simulink model "pmsm_model_Lab3_MTPA_st_R2020a"  (R2023a)
settings: Solver=ode45  StartTime=0.0  StopTime=Tf  FixedStep=Tsim  MaxStep=Tsim  MinStep=Tsim/100  RelTol=1e-3
values from neighbouring files (symbols this model uses):
  C32 = [ 1       0 ... (first row only)    [pmsm_param_Lab1_2025.m]    (also in pmsm_param_Lab2_2025_st.m; pmsm_param_Lab3_st.m; pmsm_param_Lab4_2024_st.m)
  C32inv = 2/3*[1    -1/2        -1/2 ... (first row only)    [pmsm_param_Lab1_2025.m]    (also in pmsm_param_Lab2_2025_st.m; pmsm_param_Lab3_st.m; pmsm_param_Lab4_2024_st.m)
  C33 = C32*C32inv    [pmsm_param_Lab1_2025.m]    (also in pmsm_param_Lab2_2025_st.m; pmsm_param_Lab3_st.m; pmsm_param_Lab4_2024_st.m)
  Cb = 500e-6    (= 0.0005)    [pmsm_param_Lab3_st.m]    (also in pmsm_param_Lab4_2024_st.m)
  dTm0 = 0.20*Tmrated    (= 48)    [pmsm_param_Lab2_2025_st.m]    (also in pmsm_param_Lab3_st.m; pmsm_param_Lab4_2024_st.m = 120)
  Dyno = 1    [pmsm_param_Lab3_st.m]    (also in pmsm_param_Lab4_2024_st.m = 0)
  f = 15e-3    (= 0.015)    [pmsm_param_Lab1_2025.m]    (also in pmsm_param_Lab2_2025_st.m; pmsm_param_Lab3_st.m; pmsm_param_Lab4_2024_st.m)
  GVSI = 1    [pmsm_param_Lab2_2025_st.m]    (also in pmsm_param_Lab3_st.m; pmsm_param_Lab4_2024_st.m)
  Id0 = 0    [pmsm_param_Lab1_2025.m]    (also in pmsm_param_Lab2_2025_st.m; pmsm_param_Lab3_st.m = interp1(Tref,Idopt,Tm0); pmsm_param_Lab4_2024_st.m = interp1(Tref,Idopt,Tm0))
  Idc0 = Pe0/VDC    [pmsm_param_Lab3_st.m]    (also in pmsm_param_Lab4_2024_st.m)
  Idopt = zeros(1,NT)    [pmsm_param_Lab3_st.m]    (also in pmsm_param_Lab4_2024_st.m)
  Iq0 = 2/3*Tm0/(Pp*Psif)    (= 0)    [pmsm_param_Lab1_2025.m]    (also in pmsm_param_Lab2_2025_st.m = 119.926066866; pmsm_param_Lab3_st.m = interp1(Tref,Iqopt,Tm0); pmsm_param_Lab4_2024_st.m = interp1(Tref,Iqopt,Tm0))
  Iqopt = zeros(1,NT)    [pmsm_param_Lab3_st.m]    (also in pmsm_param_Lab4_2024_st.m)
  J = 100e-3    (= 0.1)    [pmsm_param_Lab1_2025.m]    (also in pmsm_param_Lab2_2025_st.m; pmsm_param_Lab3_st.m; pmsm_param_Lab4_2024_st.m)
  Kid = Kpd / tid    (= 282.743237724)    [pmsm_param_Lab2_2025_st.m]    (also in pmsm_param_Lab3_st.m = 180; pmsm_param_Lab4_2024_st.m = 180)
  Kiq = Kpq / tiq    (= 282.743237724)    [pmsm_param_Lab2_2025_st.m]    (also in pmsm_param_Lab3_st.m = 180; pmsm_param_Lab4_2024_st.m = 180)
  kL = 0.750    (= 0.75)    [pmsm_param_Lab1_2025.m]    (also in pmsm_param_Lab2_2025_st.m; pmsm_param_Lab3_st.m; pmsm_param_Lab4_2024_st.m)
  Kpd = (3*Ld0) / tr    (= 6.28318306054)    [pmsm_param_Lab2_2025_st.m]    (also in pmsm_param_Lab3_st.m = 3; pmsm_param_Lab4_2024_st.m = 3)
  Kpq = (3 * Lq0) / tr    (= 3.14159153027)    [pmsm_param_Lab2_2025_st.m]    (also in pmsm_param_Lab3_st.m = 6; pmsm_param_Lab4_2024_st.m = 6)
  Lb = 20e-6    (= 2e-05)    [pmsm_param_Lab3_st.m]    (also in pmsm_param_Lab4_2024_st.m)
  Ld0 = 2.0*Ld    (= 0.002)    [pmsm_param_Lab2_2025_st.m]    (also in pmsm_param_Lab3_st.m = 0.001; pmsm_param_Lab4_2024_st.m = 0.001)
  Lq0 = 0.5*Lq    (= 0.001)    [pmsm_param_Lab2_2025_st.m]    (also in pmsm_param_Lab3_st.m = 0.002; pmsm_param_Lab4_2024_st.m = 0.002)
  Pe0 = 3/2*(Vd0*Id0+Vq0*Iq0)    [pmsm_param_Lab2_2025_st.m]    (also in pmsm_param_Lab3_st.m; pmsm_param_Lab4_2024_st.m)
  Pp = 4    [pmsm_param_Lab1_2025.m]    (also in pmsm_param_Lab2_2025_st.m; pmsm_param_Lab3_st.m; pmsm_param_Lab4_2024_st.m)
  Psid0 = interpn(Idv,Iqv,Psidd,Id0,Iq0)    [pmsm_param_Lab1_2025.m]    (also in pmsm_param_Lab2_2025_st.m; pmsm_param_Lab3_st.m; pmsm_param_Lab4_2024_st.m)
  Psif0 = 1.0*Psif    (= 0.167)    [pmsm_param_Lab2_2025_st.m]    (also in pmsm_param_Lab3_st.m; pmsm_param_Lab4_2024_st.m)
  Psiq0 = interpn(Idv,Iqv,Psiqq,Id0,Iq0)    [pmsm_param_Lab1_2025.m]    (also in pmsm_param_Lab2_2025_st.m; pmsm_param_Lab3_st.m; pmsm_param_Lab4_2024_st.m)
  Qbat = 72*3600    (= 259200)    [pmsm_param_Lab3_st.m]    (also in pmsm_param_Lab4_2024_st.m)
  RateTm = 10000    [pmsm_param_Lab3_st.m]    (also in pmsm_param_Lab4_2024_st.m)
  rb = 80e-3    (= 0.08)    [pmsm_param_Lab3_st.m]    (also in pmsm_param_Lab4_2024_st.m)
  Rs = 60e-3    (= 0.06)    [pmsm_param_Lab1_2025.m]    (also in pmsm_param_Lab2_2025_st.m; pmsm_param_Lab3_st.m; pmsm_param_Lab4_2024_st.m)
  Rs0 = 1.5*Rs    (= 0.09)    [pmsm_param_Lab2_2025_st.m]    (also in pmsm_param_Lab3_st.m = 0.06; pmsm_param_Lab4_2024_st.m = 0.06)
  SOC0 = 0.50    (= 0.5)    [pmsm_param_Lab3_st.m]    (also in pmsm_param_Lab4_2024_st.m)
  Thetae0 = 0    [pmsm_param_Lab1_2025.m]    (also in pmsm_param_Lab2_2025_st.m; pmsm_param_Lab3_st.m; pmsm_param_Lab4_2024_st.m)
  Tm0 = (kL+f)*Wm0    (= 0)    [pmsm_param_Lab1_2025.m]    (also in pmsm_param_Lab2_2025_st.m = 120.165919; pmsm_param_Lab3_st.m = 192.2654704; pmsm_param_Lab4_2024_st.m)
  Tp = 100e-6    (= 0.0001)    [pmsm_param_Lab2_2025_st.m]    (also in pmsm_param_Lab3_st.m; pmsm_param_Lab4_2024_st.m)
  Tref = -Tmax:Tmax/100:Tmax    [pmsm_param_Lab3_st.m]    (also in pmsm_param_Lab4_2024_st.m)
  Ts = Tsim    [pmsm_param_Lab2_2025_st.m]    (also in pmsm_param_Lab3_st.m = 0.0001; pmsm_param_Lab4_2024_st.m = 0.0001)
  Tsim = 1e-6    (= 1e-06)    [pmsm_param_Lab1_2025.m]    (also in pmsm_param_Lab2_2025_st.m = min([Tp Ts])/100; pmsm_param_Lab3_st.m = min([Tp Ts])/100; pmsm_param_Lab4_2024_st.m = min([Tp Ts])/100)
  TSS = Tstep+0.050    (= 0.1)    [pmsm_param_Lab3_st.m]    (also in pmsm_param_Lab4_2024_st.m)
  Tstep = 0.10    (= 0.1)    [pmsm_param_Lab2_2025_st.m]    (also in pmsm_param_Lab3_st.m = 0.05; pmsm_param_Lab4_2024_st.m = 0.05)
  Ud0 = Rs*Id0    (= 0)    [pmsm_param_Lab2_2025_st.m]    (also in pmsm_param_Lab3_st.m; pmsm_param_Lab4_2024_st.m)
  Uq0 = Rs*Iq0    (= 7.19556401196)    [pmsm_param_Lab2_2025_st.m]    (also in pmsm_param_Lab3_st.m = 11.5129024191; pmsm_param_Lab4_2024_st.m = Rs*Iq0)
  Vd0 = Rs*Id0-Pp*Psiq0*Wm0    [pmsm_param_Lab1_2025.m]    (also in pmsm_param_Lab2_2025_st.m = Ud0-Pp*Psiq0*Wm0; pmsm_param_Lab3_st.m = Ud0-Pp*Psiq0*Wm0; pmsm_param_Lab4_2024_st.m = Ud0-Pp*Psiq0*Wm0)
  VDC = 800    [pmsm_param_Lab2_2025_st.m]    (also in pmsm_param_Lab3_st.m; pmsm_param_Lab4_2024_st.m)
  VDC0 = 0.8*VDC    (= 640)    [pmsm_param_Lab3_st.m]    (also in pmsm_param_Lab4_2024_st.m)
  Vp = VDC/2    (= 400)    [pmsm_param_Lab2_2025_st.m]    (also in pmsm_param_Lab3_st.m; pmsm_param_Lab4_2024_st.m)
  Vq0 = Rs*Iq0+Pp*Psid0*Wm0    [pmsm_param_Lab1_2025.m]    (also in pmsm_param_Lab2_2025_st.m = Uq0+Pp*Psid0*Wm0; pmsm_param_Lab3_st.m = Uq0+Pp*Psid0*Wm0; pmsm_param_Lab4_2024_st.m = Uq0+Pp*Psid0*Wm0)
  Wm0 = 0    [pmsm_param_Lab1_2025.m]    (also in pmsm_param_Lab2_2025_st.m = 157.079632679; pmsm_param_Lab3_st.m = 251.327412287; pmsm_param_Lab4_2024_st.m)
undefined symbols (not defined in the file or in its folder): Idd, Idrop, Iqq, Isw, Psidv, Psiqv, SwLoss, Vdrop
libraries: simulink x11, spsTHDLib x1
(part 1 of 2)
settings Model: Creator=babak_  LastModifiedBy=Henry
settings SolverCC: AlgebraicLoopSolver=LineSearch
settings DataIOCC: LimitDataPoints=on  SaveFormat=Array  SignalLoggingSaveFormat=ModelDataLogs  ReturnWorkspaceOutputs=off
settings OptimizationCC: BooleanDataType=off  ExpressionDepthLimit=2147483647  InitFltsAndDblsToZero=on  LifeSpan=inf
settings DebuggingCC: SaveWithParameterizedLinksMsg=none  UnderspecifiedInitializationDetection=Classic  MergeDetectMultiDrivingBlocksExec=none  SignalResolutionControl=TryResolveAllWithWarning  MultiTaskDSMMsg=warning  MultiTaskCondExecSysMsg=none  FcnCallInpInsideContextMsg=warning  UnconnectedInputMsg=warning  UnconnectedOutputMsg=warning  UnconnectedLineMsg=warning  StateNameClashWarn=warning  SFUnexpectedBacktrackingDiag=warning  SFNoUnconditionalDefaultTransitionDiag=warning  ArithmeticOperatorsInVariantConditions=warning
settings HardwareCC: ProdBitPerPointer=32  ProdBitPerSizeT=32  ProdBitPerPtrDiffT=32  ProdLargestAtomicFloat=None  ProdIntDivRoundTo=Undefined  ProdEndianess=Unspecified  ProdWordSize=32  ProdHWDeviceType=32-bit Generic  TargetUnknown=on
settings ModelReferenceCC: EnableRefExpFcnMdlSchedulingChecks=on  PropagateSignalLabelsOutOfModel=off
settings SFSimCC: SimUseLocalCustomCode=off  CustomCodeUndefinedFunction=UseInterfaceOnly
settings RTWCC: RTWUseLocalCustomCode=off
settings CodeAppCC: StateflowObjectComments=on
settings GRTTargetCC: TargetFcnLib=ansi_tfl_tmw.mat  TargetLangStandard=C89/C90 (ANSI)  ModelReferenceCompliant=off  CompOptLevelCompliant=off  CombineOutputUpdateFcns=off  MatFileLogging=off  GRTInterface=on
settings ConfigComp: CovMetricSettings=dw  CovSaveCumulativeToWorkspaceVar=on  CovSaveSingleToWorkspaceVar=on  CovExternalEMLEnable=off

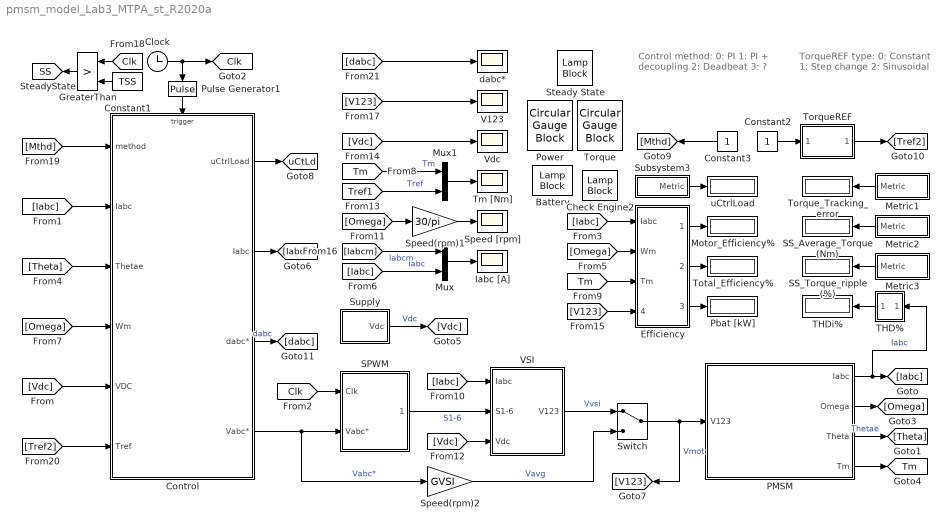
== system pmsm_model_Lab3_MTPA_st_R2020a ==
  note: Control method:
      | 0: PI
      | 1: PI + decoupling
      | 2: Deadbeat
      | 3: ?
  note: TorqueREF type:
      | 0: Constant
      | 1: Step change
      | 2: Sinusoidal
  "            SS_Average_Torque (Nm)" : Display
  "      Torque_Tracking_error" : Display
  "     SS_Torque_ripple (%)" : Display
  Battery : LampBlock  LabelPosition=Hide  Icon=Battery
  Check Engine2 : LampBlock  LabelPosition=Hide  Icon=CheckEngine2
  Clock : Clock
  Constant1 : Constant  Value=TSS
  Constant2 : Constant
  Constant3 : Constant
  Control : Subsystem
  Efficiency : Subsystem
  GreaterThan : RelationalOperator  Operator=>  RndMeth=Round  InputSameDT=off
  Iabc [A] : Scope
  Metric1 : Subsystem
  Metric2 : Subsystem
  Metric3 : Subsystem
  Motor_Efficiency% : Display
  Mux : Mux  Inputs=2
  Mux1 : Mux  Inputs=2
  PMSM : Subsystem
  Pbat [kW] : Display
  Power : CircularGaugeBlock  LabelPosition=Hide  ScaleMin=-20
  Pulse Generator1 : DiscretePulseGenerator  PulseType=Time based  TimeSource=Use external signal  Period=Ts  PhaseDelay=Tsim
  SPWM : Subsystem
  Speed [rpm] : Scope
  Speed(rpm)1 : Gain  Gain=30/pi
  Speed(rpm)2 : Gain  Gain=GVSI
  Steady State : LampBlock  LabelPosition=Hide
  Subsystem3 : Subsystem
  Supply : Subsystem
      settings: PortSchema="{\"entries\":[{\"content\":{\"sides\":[{\"content\":{},\"type\":\"ConnectorPlacement.EquallySpacedRectSide\",\"uuid\":\"f6a50b0e-e406-44ec-a837-188ccf25c988\"},{\"content\":{\"side\":\"RIGHT\"},\"type\":\"ConnectorPlacement.EquallySpacedRectSide\",\"uuid\":\"758525d2-b429-4a35-a56f-d60ac10ca8a9\"},{\"content\":{\"connectorIds\":[\"Out1\"],\"side\":\"TOP\"},\"type\":\"ConnectorPlacement.EquallySpacedRectSide\",\"uuid\":\"bedbcc07-640a-4a94-abcb-a05396b336d1\"}]},\"type\":\"ConnectorPlacement.EquallySpacedConnector\",\"uuid\":\"fd90f98a-c249-4d99-b745-2239d5baaabe\"}],\"packageUris\":[\"http://schema.mathworks.com/mf0/Connector/R2020b\"],\"version\":\"1.0\"}"
  Switch : ManualSwitch
  THD% : Subsystem
  THDi% : Display
  Tm [Nm] : Scope
  Torque : CircularGaugeBlock  LabelPosition=Hide  ScaleMax=300
  TorqueREF : Subsystem
  "Total_Efficiency% " : Display
  "V123 " : Scope
  VSI : Subsystem
  Vdc : Scope
  dabc* : Scope
  uCtrlLoad : Display
  tag scope: Clk=global, SS=global, Tm=global, uCtLd=global
  wires:
  PMSM/3(Theta) -> [Theta]  "Thetae"
  PMSM/4(Tm) -> [Tm]
  Clock/1 -> [Clk], Pulse Generator1/1
  PMSM/1(Iabc) -> [Iabc], THD%/1(Iabc)  "Iabc"
  [Iabc] -> Control/2(Iabc)
  PMSM/2(Omega) -> [Omega]
  [Theta] -> Control/3(Thetae)
  [Omega] -> Control/4(Wm)
  Supply/1("Vdc ") -> [Vdc]  "Vdc"
  SPWM/1(pulses) -> VSI/2(S1-6)  "S1-6"
  [Iabc] -> VSI/1(Iabc)
  [Clk] -> SPWM/1(Clk)
  VSI/1(V123) -> Switch/1  "Vvsi"
  [Iabc] -> Efficiency/1(Iabc)
  Efficiency/1(etaMot) -> Motor_Efficiency%/1
  [Tm] -> Efficiency/3(Tm)
  [Omega] -> Efficiency/2(Wm)
  Efficiency/2(etaTot) -> "Total_Efficiency% "/1
  Metric1/1("Metric ") -> "      Torque_Tracking_error"/1
  Metric2/1(Metric) -> "            SS_Average_Torque (Nm)"/1
  Metric3/1(Metric) -> "     SS_Torque_ripple (%)"/1
  Speed(rpm)1/1 -> Speed [rpm]/1
  [Omega] -> Speed(rpm)1/1
  [Clk] -> GreaterThan/1
  [Iabc] -> Mux/2  "`Iabc"
  Constant1/1 -> GreaterThan/2
  GreaterThan/1 -> [SS]
  THD%/1(" ") -> THDi%/1
  Control/4(Vabc*) -> SPWM/2(Vabc*), Speed(rpm)2/1  "Vabc*"
  [Vdc] -> Control/5(VDC)
  [Vdc] -> VSI/3(Vdc)
  [Mthd] -> Control/1(method)
  Switch/1 -> PMSM/1(V123), [V123]  "Vmot"
  Pulse Generator1/1 -> Control/Trigger
  Speed(rpm)2/1 -> Switch/2  "Vavg"
  Efficiency/3(Pbat) -> Pbat [kW]/1
  [Tref2] -> Control/6(Tref)
  Control/3(dabc*) -> [dabc]  "dabc"
  [Vdc] -> Vdc/1
  Control/2("Iabc ") -> [Iabcm]
  Mux/1 -> Iabc [A]/1
  [Iabcm] -> Mux/1  "Iabcm"
  Subsystem3/1(Metric) -> uCtrlLoad/1
  Control/1(uCtrlLoad) -> [uCtLd]
  [V123] -> Efficiency/4(V123)
  [V123] -> "V123 "/1
  Mux1/1 -> Tm [Nm]/1
  [Tm] -> Mux1/1  "Tm"
  [Tref1] -> Mux1/2  "Tref"
  Constant3/1 -> [Mthd]
  TorqueREF/1(Tref2) -> [Tref2]
  Constant2/1 -> TorqueREF/1(Type)
  [dabc] -> dabc*/1

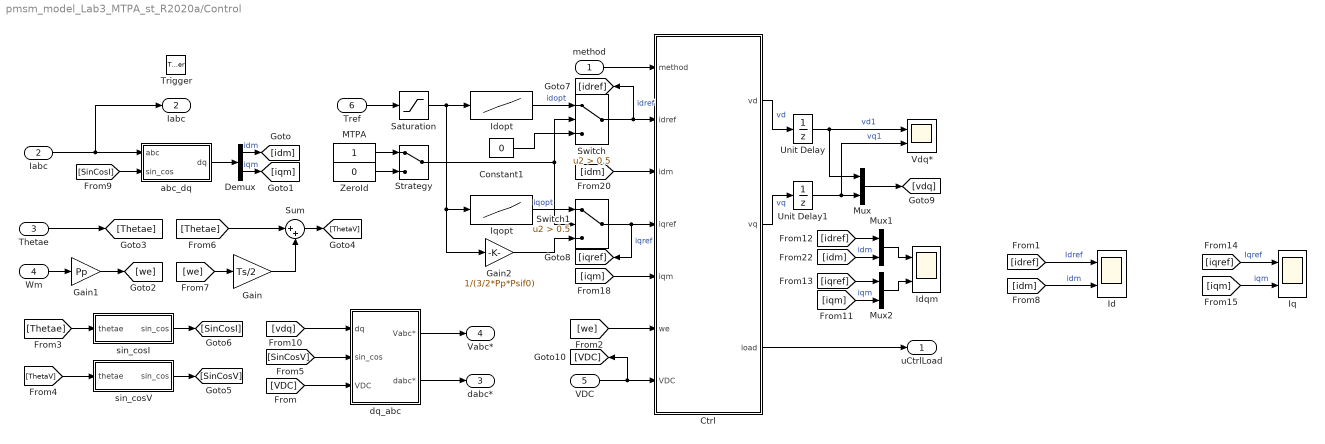
== system pmsm_model_Lab3_MTPA_st_R2020a/Control ==
  method : Inport
  Iabc : Inport  Port=2
  Thetae : Inport  Port=3
  Wm : Inport  Port=4
  VDC : Inport  Port=5
  Tref : Inport  Port=6
  Trigger : TriggerPort  TriggerType=falling  VariantControl=Variant  PortDimensions=1
  Constant1 : Constant  Value=0
  Ctrl : MATLAB Function  TreatAsAtomicUnit=on
  Demux : Demux  Outputs=2
  Gain : Gain  Gain=Ts/2
  Gain1 : Gain  Gain=Pp
  Gain2 : Gain  Gain=1/(3/2*Pp*Psif0)
  Id : Scope  NumInputPorts=2
  Idopt : Lookup_n-D  NumberOfTableDimensions=1  BreakpointsForDimension1=Tref  Table=Idopt  InternalRulePriority=Speed  RndMeth=Simplest
  Idqm : Scope  NumInputPorts=2
  Iq : Scope  NumInputPorts=2
  Iqopt : Lookup_n-D  NumberOfTableDimensions=1  BreakpointsForDimension1=Tref  Table=Iqopt  InternalRulePriority=Speed  RndMeth=Simplest
  MTPA : Constant
  Mux : Mux  Inputs=2
  Mux1 : Mux  Inputs=2
  Mux2 : Mux  Inputs=2
  Saturation : Saturate  UpperLimit=max(Tref)  LowerLimit=min(Tref)
  Strategy : ManualSwitch
  Sum : Sum  Inputs=|++
  Switch : Switch  Criteria=u2 > Threshold  Threshold=0.5  SaturateOnIntegerOverflow=off  InputSameDT=off
  Switch1 : Switch  Criteria=u2 > Threshold  Threshold=0.5  SaturateOnIntegerOverflow=off  InputSameDT=off
  Unit Delay : UnitDelay  InitialCondition=Vd0  SampleTime=-1  HasFrameUpgradeWarning=on
  Unit Delay1 : UnitDelay  InitialCondition=Vq0  SampleTime=-1  HasFrameUpgradeWarning=on
  Vdq* : Scope  NumInputPorts=2
  ZeroId : Constant  Value=0
  abc_dq : Subsystem
  dq_abc : Subsystem
  sin_cosI : Subsystem
  sin_cosV : Subsystem
  uCtrlLoad : Outport
  "Iabc " : Outport  Port=2
  dabc* : Outport  Port=3
  Vabc* : Outport  Port=4
  wires:
  [SinCosI] -> abc_dq/2(sin_cos)
  sin_cosI/1(sin_cos) -> [SinCosI]
  [SinCosV] -> dq_abc/2(sin_cos)
  Ctrl/2(vq) -> Unit Delay1/1  "vq"
  Ctrl/1(vd) -> Unit Delay/1  "vd"
  [Thetae] -> sin_cosI/1(thetae)
  [ThetaV] -> sin_cosV/1(thetae)
  sin_cosV/1(sin_cos) -> [SinCosV]
  Sum/1 -> [ThetaV]
  [Thetae] -> Sum/1
  [we] -> Gain/1
  Gain/1 -> Sum/2
  Iabc/1 -> "Iabc "/1, abc_dq/1(abc)
  Gain1/1 -> [we]
  [iqm] -> Mux2/2  "iqm"
  Demux/1 -> [idm]  "idm"
  [idm] -> Mux1/2  "idm"
  Demux/2 -> [iqm]  "iqm"
  Mux2/1 -> Idqm/2
  Mux1/1 -> Idqm/1
  abc_dq/1(dq) -> Demux/1
  Mux/1 -> [vdq]
  [vdq] -> dq_abc/1(dq)
  Wm/1 -> Gain1/1
  Thetae/1 -> [Thetae]
  [idref] -> Mux1/1
  [iqref] -> Mux2/1
  dq_abc/1(Vabc*) -> Vabc*/1
  [idm] -> Ctrl/3(idm)
  [we] -> Ctrl/6(we)
  [iqm] -> Ctrl/5(iqm)
  method/1 -> Ctrl/1(method)
  Idopt/1 -> Switch/1  "idopt"
  Iqopt/1 -> Switch1/1  "iqopt"
  Tref/1 -> Saturation/1
  Unit Delay/1 -> Mux/1, Vdq*/1  "vd1"
  Unit Delay1/1 -> Mux/2, Vdq*/2  "vq1"
  VDC/1 -> [VDC], Ctrl/7(VDC)
  Ctrl/3(load) -> uCtrlLoad/1
  dq_abc/2(dabc*) -> dabc*/1
  [VDC] -> dq_abc/3(VDC)
  Switch/1 -> [idref], Ctrl/2(idref)  "idref"
  Switch1/1 -> [iqref], Ctrl/4(iqref)  "iqref"
  Strategy/1 -> Switch/2, Switch1/2
  Gain2/1 -> Switch1/3
  MTPA/1 -> Strategy/1
  ZeroId/1 -> Strategy/2
  Constant1/1 -> Switch/3
  Saturation/1 -> Gain2/1, Iqopt/1, Idopt/1
  [idref] -> Id/1  "Idref"
  [idm] -> Id/2  "idm"
  [iqref] -> Iq/1  "Iqref"
  [iqm] -> Iq/2  "iqm"

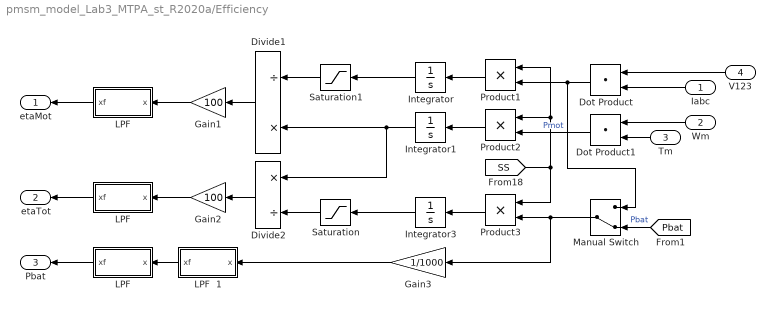
== system pmsm_model_Lab3_MTPA_st_R2020a/Efficiency ==
  Iabc : Inport
  Wm : Inport  Port=2
  Tm : Inport  Port=3
  V123 : Inport  Port=4
  Divide1 : Product  Inputs=/*
  Divide2 : Product  Inputs=*/
  Dot Product : DotProduct  OutDataTypeStr=Inherit: Inherit via internal rule
  Dot Product1 : DotProduct  OutDataTypeStr=Inherit: Inherit via internal rule
  Gain1 : Gain  Gain=100
  Gain2 : Gain  Gain=100
  Gain3 : Gain  Gain=1/1000
  Integrator : Integrator  InitialCondition=1
  Integrator1 : Integrator
  Integrator3 : Integrator  InitialCondition=1
  LPF : Subsystem
  "LPF " : Subsystem
  "LPF  " : Subsystem
  LPF  1 : Subsystem
  Manual Switch : ManualSwitch  CurrentSetting=0
  Product1 : Product
  Product2 : Product
  Product3 : Product
  Saturation : Saturate  UpperLimit=inf  LowerLimit=1
  Saturation1 : Saturate  UpperLimit=inf  LowerLimit=1
  etaMot : Outport
  etaTot : Outport  Port=2
  Pbat : Outport  Port=3
  wires:
  Dot Product/1 -> Product1/2, Manual Switch/1  "Pmot"
  Dot Product1/1 -> Product2/2
  Wm/1 -> Dot Product1/1
  V123/1 -> Dot Product/1
  Tm/1 -> Dot Product1/2
  Iabc/1 -> Dot Product/2
  Integrator1/1 -> Divide2/1, Divide1/2
  Gain1/1 -> LPF/1(x)
  Divide1/1 -> Gain1/1
  Divide2/1 -> Gain2/1
  Gain2/1 -> "LPF "/1(x)
  Saturation/1 -> Divide2/2
  [Pbat] -> Manual Switch/2  "Pbat"
  Integrator/1 -> Saturation1/1
  LPF/1(xf) -> etaMot/1
  "LPF "/1(xf) -> etaTot/1
  Integrator3/1 -> Saturation/1
  Product1/1 -> Integrator/1
  Product2/1 -> Integrator1/1
  Product3/1 -> Integrator3/1
  [SS] -> Product3/1, Product1/1, Product2/1
  Saturation1/1 -> Divide1/1
  Manual Switch/1 -> Gain3/1, Product3/2
  "LPF  "/1(xf) -> Pbat/1
  Gain3/1 -> LPF  1/1(x)
  LPF  1/1(xf) -> "LPF  "/1(x)

== system pmsm_model_Lab3_MTPA_st_R2020a/Metric1 ==
  Demux : Demux  Outputs=2
  ITSE : Subsystem
  LPF : Subsystem
  Multiport Switch1 : MultiPortSwitch  DataPortOrder=Zero-based contiguous  Inputs=4  zeroidx=on  SaturateOnIntegerOverflow=off  InputSameDT=off
  RMSE : Subsystem
  Sum : Sum  Inputs=+-|
  "Metric " : Outport
  wires:
  Demux/1 -> Sum/1  "Tref"
  [Tm] -> Sum/2  "Tm"
  Sum/1 -> RMSE/1(Err), ITSE/1(Err)  "Terr"
  [Tref] -> Demux/1
  Demux/2 -> Multiport Switch1/1
  Multiport Switch1/1 -> LPF/1(x)
  RMSE/1(RMSE) -> Multiport Switch1/2, Multiport Switch1/4, Multiport Switch1/5
  ITSE/1(Metric) -> Multiport Switch1/3
  LPF/1(xf) -> "Metric "/1  "Ttrack"

== system pmsm_model_Lab3_MTPA_st_R2020a/Metric2 ==
  LPF : Subsystem
  Window : Subsystem
  Metric : Outport
  wires:
  Window/1(Tav) -> Metric/1  "Tav"
  [Tm] -> LPF/1(Tm)
  LPF/1(Tav) -> Window/1("Tav ")

== system pmsm_model_Lab3_MTPA_st_R2020a/Metric3 ==
  Constant : Constant  Value=0
  Demux : Demux  Outputs=2
  LPF : Subsystem
  LPF2 : Subsystem
  Multiport Switch : MultiPortSwitch  DataPortOrder=Zero-based contiguous  Inputs=4  zeroidx=on  SaturateOnIntegerOverflow=off  InputSameDT=off
  Ripple : Subsystem
  Terminator : Terminator
  Metric : Outport
  wires:
  LPF/1(Tmh) -> Ripple/1(Tmh)
  [Tm] -> LPF/1(Tm)
  [Tref] -> Demux/1
  Multiport Switch/1 -> LPF2/1(x)
  Demux/2 -> Multiport Switch/1
  Demux/1 -> Terminator/1
  Constant/1 -> Multiport Switch/4, Multiport Switch/5
  Ripple/1(Ripple) -> Multiport Switch/2, Multiport Switch/3
  LPF/2(Tm0) -> Ripple/2(Tm0)
  LPF2/1(xf) -> Metric/1  "Tripple"

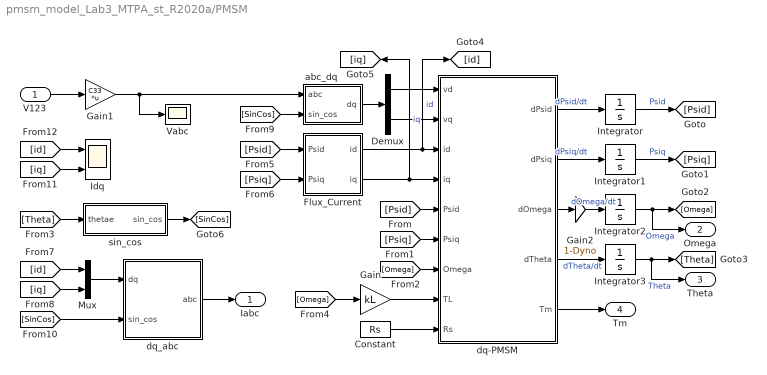
== system pmsm_model_Lab3_MTPA_st_R2020a/PMSM ==
  V123 : Inport
  Constant : Constant  Value=Rs
  Demux : Demux  Outputs=2
  Flux_Current : Subsystem
  Gain : Gain  Gain=kL
  Gain1 : Gain  Gain=C33  Multiplication=Matrix(K*u)
  Gain2 : Gain  Gain=1-Dyno
  Idq : Scope  NumInputPorts=2
  Integrator : Integrator  InitialCondition=Psid0
  Integrator1 : Integrator  InitialCondition=Psiq0
  Integrator2 : Integrator  InitialCondition=Wm0
  Integrator3 : Integrator  InitialCondition=Thetae0
  Mux : Mux  Inputs=2
  Vabc : Scope
  abc_dq : Subsystem
  dq-PMSM : MATLAB Function  TreatAsAtomicUnit=on
  dq_abc : Subsystem
  sin_cos : Subsystem
  Iabc : Outport
  Omega : Outport  Port=2
  Theta : Outport  Port=3
  Tm : Outport  Port=4
  wires:
  dq-PMSM/1(dPsid) -> Integrator/1  "dPsid/dt"
  dq-PMSM/2(dPsiq) -> Integrator1/1  "dPsiq/dt"
  Integrator3/1 -> [Theta], Theta/1  "Theta"
  [Omega] -> Gain/1
  Flux_Current/1(id) -> [id], dq-PMSM/3(id)  "id"
  [SinCos] -> dq_abc/2(sin_cos)
  Integrator1/1 -> [Psiq]  "Psiq"
  sin_cos/1(sin_cos) -> [SinCos]
  dq_abc/1(abc) -> Iabc/1
  dq-PMSM/4(dTheta) -> Integrator3/1  "dTheta/dt"
  Demux/1 -> dq-PMSM/1(vd)
  [iq] -> Mux/2
  Mux/1 -> dq_abc/1(dq)
  dq-PMSM/3(dOmega) -> Gain2/1
  [Psiq] -> dq-PMSM/6(Psiq)
  [Psid] -> dq-PMSM/5(Psid)
  [Theta] -> sin_cos/1(thetae)
  abc_dq/1(dq) -> Demux/1
  [SinCos] -> abc_dq/2(sin_cos)
  Gain/1 -> dq-PMSM/8(TL)
  Demux/2 -> dq-PMSM/2(vq)
  [Omega] -> dq-PMSM/7(Omega)
  V123/1 -> Gain1/1
  [id] -> Mux/1
  Integrator2/1 -> [Omega], Omega/1  "Omega"
  Flux_Current/2(iq) -> dq-PMSM/4(iq), [iq]  "iq"
  Integrator/1 -> [Psid]  "Psid"
  Constant/1 -> dq-PMSM/9(Rs)
  Gain1/1 -> abc_dq/1(abc), Vabc/1
  dq-PMSM/5(Tm) -> Tm/1
  [id] -> Idq/1
  [iq] -> Idq/2
  [Psid] -> Flux_Current/1(Psid)
  [Psiq] -> Flux_Current/2(Psiq)
  Gain2/1 -> Integrator2/1  "dOmega/dt"

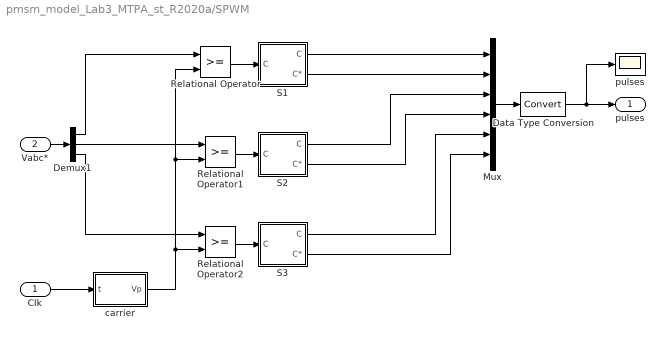
== system pmsm_model_Lab3_MTPA_st_R2020a/SPWM ==
  Clk : Inport
  Vabc* : Inport  Port=2
  Data Type Conversion : DataTypeConversion  SaturateOnIntegerOverflow=off  RndMeth=Floor
  Demux1 : Demux  Outputs=3
      settings: DisplayOption=none
  Mux : Mux  Inputs=6
  Relational Operator : RelationalOperator  OutDataTypeStr=boolean
  Relational Operator1 : RelationalOperator  OutDataTypeStr=boolean
  Relational Operator2 : RelationalOperator  OutDataTypeStr=boolean
  S1 : Subsystem
  S2 : Subsystem
  S3 : Subsystem
  carrier : Subsystem
  "pulses " : Scope
  pulses : Outport  InitialOutput=0
  wires:
  Mux/1 -> Data Type Conversion/1
  Clk/1 -> carrier/1(t)
  Relational Operator/1 -> S1/1("C ")
  Relational Operator1/1 -> S2/1("C ")
  Relational Operator2/1 -> S3/1("C ")
  Vabc*/1 -> Demux1/1
  Demux1/1 -> Relational Operator/1
  Demux1/2 -> Relational Operator1/1
  Demux1/3 -> Relational Operator2/1
  S1/1(C) -> Mux/1
  S1/2(C*) -> Mux/2
  S2/1(C) -> Mux/3
  S2/2(C*) -> Mux/4
  S3/1(C) -> Mux/5
  S3/2(C*) -> Mux/6
  Data Type Conversion/1 -> "pulses "/1, pulses/1
  carrier/1(Vp) -> Relational Operator2/2, Relational Operator1/2, Relational Operator/2

== system pmsm_model_Lab3_MTPA_st_R2020a/Subsystem3 ==
  Divide : Product  Inputs=/*
  Saturation : Saturate  UpperLimit=inf  LowerLimit=1e-3
  Metric : Outport
  wires:
  Saturation/1 -> Divide/1
  [Clk] -> Saturation/1
  [uCtLd] -> Divide/2
  Divide/1 -> Metric/1

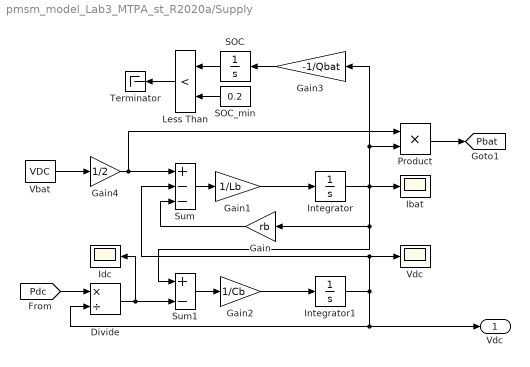
== system pmsm_model_Lab3_MTPA_st_R2020a/Supply ==
  Divide : Product  Inputs=*/
  Gain : Gain  Gain=rb
  Gain1 : Gain  Gain=1/Lb
  Gain2 : Gain  Gain=1/Cb
  Gain3 : Gain  Gain=-1/Qbat
  Gain4 : Gain  Gain=1/2
  Ibat : Scope
  Idc : Scope
  Integrator : Integrator  InitialCondition=Idc0
  Integrator1 : Integrator  InitialCondition=VDC  LimitOutput=on  LowerSaturationLimit=1
  Less Than : RelationalOperator  Operator=<  OutDataTypeStr=boolean  RndMeth=Simplest  InputSameDT=off
  Product : Product
  SOC : Integrator  InitialCondition=SOC0  LimitOutput=on  UpperSaturationLimit=1  LowerSaturationLimit=0
  SOC_min : Constant  Value=0.2
  Sum : Sum  Inputs=+--
  Sum1 : Sum  Inputs=+-
  Terminator : Terminator
  Vbat : Constant  Value=VDC
  Vdc : Scope
  "Vdc " : Outport
  tag scope: Pbat=global
  wires:
  Vbat/1 -> Gain4/1
  Integrator/1 -> Gain3/1, Product/2, Ibat/1, Gain/1, Sum1/1
  Gain1/1 -> Integrator/1
  Gain/1 -> Sum/3
  Gain2/1 -> Integrator1/1
  Sum1/1 -> Gain2/1
  Sum/1 -> Gain1/1
  Product/1 -> [Pbat]
  Divide/1 -> Idc/1, Sum1/2
  [Pdc] -> Divide/1
  Integrator1/1 -> "Vdc "/1, Divide/2, Sum/2, Vdc/1
  Gain3/1 -> SOC/1
  SOC_min/1 -> Less Than/2
  Less Than/1 -> Terminator/1
  SOC/1 -> Less Than/1
  Gain4/1 -> Sum/1, Product/1

== system pmsm_model_Lab3_MTPA_st_R2020a/THD% ==
  Iabc : Inport
  Product : Product
  THD : spsTHDLib/THD  Freq=Wm0*Pp/2/pi  Ts=0
  percent : Gain  Gain=100*ones(1,3)/3  Multiplication=Matrix(K*u) (u vector)
  " " : Outport
  wires:
  THD/1 -> percent/1
  percent/1 -> " "/1
  Iabc/1 -> Product/1
  [SS] -> Product/2
  Product/1 -> THD/1

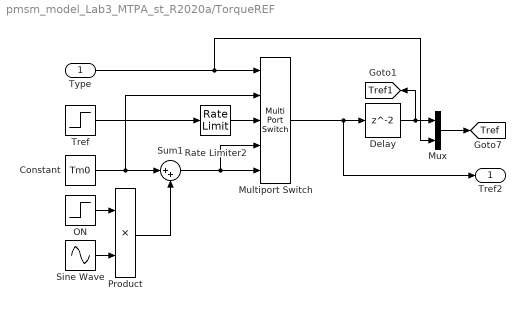
== system pmsm_model_Lab3_MTPA_st_R2020a/TorqueREF ==
  Type : Inport
  Constant : Constant  Value=Tm0  SampleTime=0
  Delay : Delay  InitialCondition=Tm0  SampleTime=Ts
  Multiport Switch : MultiPortSwitch  DataPortOrder=Zero-based contiguous  Inputs=4  zeroidx=on  SaturateOnIntegerOverflow=off  InputSameDT=off
  Mux : Mux  Inputs=2
  ON : Step  Time=Tstep  SampleTime=0
  Product : Product
  Rate Limiter2 : RateLimiter  RisingSlewLimit=RateTm  FallingSlewLimit=-RateTm  SampleTimeMode=inherited
  Sine Wave : Sin  Amplitude=dTm0  Frequency=2*pi*500  SampleTime=0
  Sum1 : Sum  Inputs=|++
  Tref : Step  Time=Tstep  Before=Tm0  After=Tm0+dTm0  SampleTime=0
  Tref2 : Outport
  tag scope: Tref1=global, Tref=global
  wires:
  ON/1 -> Product/1
  Sine Wave/1 -> Product/2
  Sum1/1 -> Multiport Switch/4, Multiport Switch/5
  Constant/1 -> Multiport Switch/2, Sum1/1
  Product/1 -> Sum1/2
  Delay/1 -> [Tref1], Mux/1
  Type/1 -> Mux/2, Multiport Switch/1
  Mux/1 -> [Tref]
  Tref/1 -> Rate Limiter2/1
  Multiport Switch/1 -> Delay/1, Tref2/1
  Rate Limiter2/1 -> Multiport Switch/3

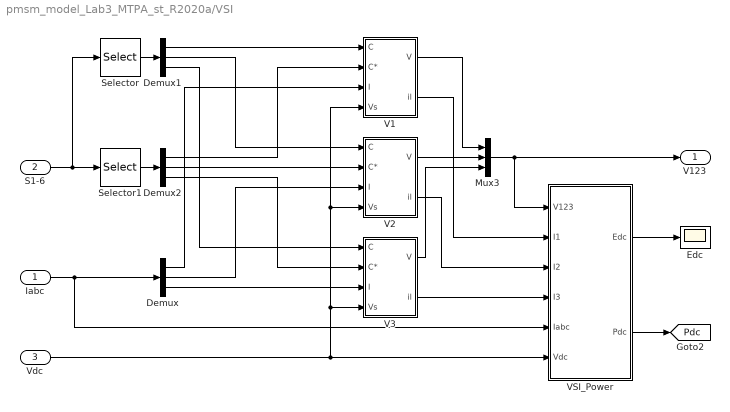
== system pmsm_model_Lab3_MTPA_st_R2020a/VSI ==
  Iabc : Inport
  S1-6 : Inport  Port=2
  Vdc : Inport  Port=3
  Demux : Demux  Outputs=3
      settings: DisplayOption=none
  Demux1 : Demux  Outputs=3
      settings: DisplayOption=none
  Demux2 : Demux  Outputs=3
      settings: DisplayOption=none
  Edc : Scope
  Mux3 : Mux  Inputs=3
  Selector : Selector  InputPortWidth=6  IndexOptions=Index vector (dialog)  Indices=[1 3 5]  OutputSizes=1
  Selector1 : Selector  InputPortWidth=6  IndexOptions=Index vector (dialog)  Indices=[2 4 6]  OutputSizes=1
  V1 : Subsystem
  V2 : Subsystem
  V3 : Subsystem
  VSI_Power : Subsystem
  V123 : Outport  InitialOutput=0
  tag scope: Pdc=global
  wires:
  V3/1(V) -> Mux3/3
  V2/1(V) -> Mux3/2
  V1/1(V) -> Mux3/1
  Iabc/1 -> Demux/1, VSI_Power/5(Iabc)
  Demux/1 -> V1/3(I)
  Demux/2 -> V2/3(I)
  Demux/3 -> V3/3(I)
  Demux2/1 -> V1/2(C*)
  Demux1/1 -> V1/1(C)
  Demux1/2 -> V2/1(C)
  Demux2/2 -> V2/2(C*)
  Demux1/3 -> V3/1(C)
  Demux2/3 -> V3/2(C*)
  Mux3/1 -> V123/1, VSI_Power/1(V123)
  Vdc/1 -> V1/4(Vs), V2/4(Vs), V3/4(Vs), VSI_Power/6(Vdc)
  S1-6/1 -> Selector/1, Selector1/1
  Selector/1 -> Demux1/1
  Selector1/1 -> Demux2/1
  VSI_Power/1(Edc) -> Edc/1
  V1/2(il) -> VSI_Power/2(I1)
  V2/2(il) -> VSI_Power/3(I2)
  V3/2(il) -> VSI_Power/4(I3)
  VSI_Power/2(Pdc) -> [Pdc]

== system pmsm_model_Lab3_MTPA_st_R2020a/Control/abc_dq ==
  abc : Inport
  sin_cos : Inport  Port=2
  Demux : Demux  Outputs=2
      settings: DisplayOption=none
  Demux1 : Demux  Outputs=2
      settings: DisplayOption=none
  Gain3 : Gain  Gain=C32inv  Multiplication=Matrix(K*u)  OutDataTypeStr=Inherit: Same as input  ParamDataTypeStr=Inherit: Same as input
  Mux : Mux  Inputs=2
  Product{,1..3} (4 alike) : Product  InputSameDT=on  RndMeth=Zero  SaturateOnIntegerOverflow=on  OutDataTypeStr=Inherit: Same as first input
  Sum : Sum  Inputs=|++  InputSameDT=on  SaturateOnIntegerOverflow=on  OutDataTypeStr=Inherit: Same as first input
  Sum1 : Sum  Inputs=|-+  InputSameDT=on  SaturateOnIntegerOverflow=on  OutDataTypeStr=Inherit: Same as first input
  dq : Outport
  wires:
  Product/1 -> Sum/1
  Product1/1 -> Sum/2
  Product2/1 -> Sum1/1
  Product3/1 -> Sum1/2
  Sum/1 -> Mux/1
  Demux/1 -> Product/1, Product2/1
  Demux1/2 -> Product/2, Product3/1
  abc/1 -> Gain3/1
  Gain3/1 -> Demux/1  "alpha_beta"
  Demux/2 -> Product1/1, Product3/2
  sin_cos/1 -> Demux1/1
  Demux1/1 -> Product1/2, Product2/2
  Mux/1 -> dq/1
  Sum1/1 -> Mux/2

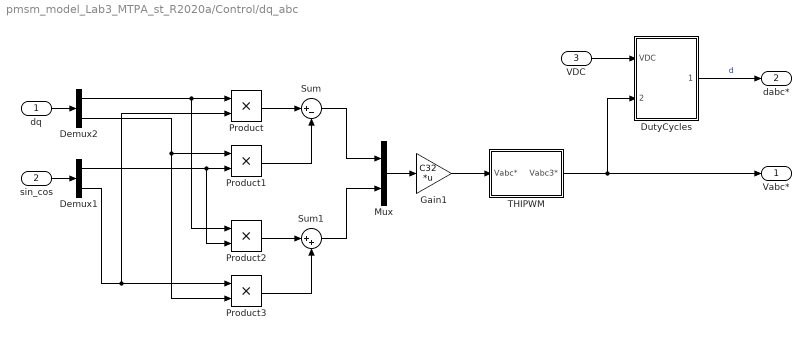
== system pmsm_model_Lab3_MTPA_st_R2020a/Control/dq_abc ==
  dq : Inport
  sin_cos : Inport  Port=2
  VDC : Inport  Port=3
  Demux1 : Demux  Outputs=2
      settings: DisplayOption=none
  Demux2 : Demux  Outputs=2
      settings: DisplayOption=none
  DutyCycles : Subsystem
  Gain1 : Gain  Gain=C32  Multiplication=Matrix(K*u)  OutDataTypeStr=Inherit: Same as input  ParamDataTypeStr=Inherit: Same as input
  Mux : Mux  Inputs=2
  Product{,1..3} (4 alike) : Product  InputSameDT=on  RndMeth=Zero  SaturateOnIntegerOverflow=on  OutDataTypeStr=Inherit: Same as first input
  Sum : Sum  Inputs=|+-  InputSameDT=on  SaturateOnIntegerOverflow=on  OutDataTypeStr=Inherit: Same as first input
  Sum1 : Sum  Inputs=|++  InputSameDT=on  SaturateOnIntegerOverflow=on  OutDataTypeStr=Inherit: Same as first input
  THIPWM : Subsystem
  Vabc* : Outport
  dabc* : Outport  Port=2
  wires:
  Gain1/1 -> THIPWM/1(Vabc*)
  Sum1/1 -> Mux/2
  Sum/1 -> Mux/1
  Demux2/2 -> Product1/1, Product3/2
  Demux2/1 -> Product2/1, Product/1
  Product/1 -> Sum/1
  Product1/1 -> Sum/2
  Product2/1 -> Sum1/1
  Product3/1 -> Sum1/2
  Demux1/2 -> Product/2, Product3/1
  sin_cos/1 -> Demux1/1
  Demux1/1 -> Product1/2, Product2/2
  Mux/1 -> Gain1/1
  dq/1 -> Demux2/1
  THIPWM/1(Vabc3*) -> DutyCycles/2(Vabc*), Vabc*/1
  VDC/1 -> DutyCycles/1(VDC)
  DutyCycles/1(dabc*) -> dabc*/1  "d"

== system pmsm_model_Lab3_MTPA_st_R2020a/Control/sin_cosI ==
  thetae : Inport
  Mux1 : Mux  Inputs=2
  Trigonometric Function : Trigonometry
  Trigonometric Function1 : Trigonometry  Operator=cos
  sin_cos : Outport
  wires:
  Mux1/1 -> sin_cos/1
  thetae/1 -> Trigonometric Function/1, Trigonometric Function1/1
  Trigonometric Function1/1 -> Mux1/2
  Trigonometric Function/1 -> Mux1/1

== system pmsm_model_Lab3_MTPA_st_R2020a/Control/sin_cosV ==
  thetae : Inport
  Mux1 : Mux  Inputs=2
  Trigonometric Function : Trigonometry
  Trigonometric Function1 : Trigonometry  Operator=cos
  sin_cos : Outport
  wires:
  Mux1/1 -> sin_cos/1
  thetae/1 -> Trigonometric Function/1, Trigonometric Function1/1
  Trigonometric Function1/1 -> Mux1/2
  Trigonometric Function/1 -> Mux1/1

== system pmsm_model_Lab3_MTPA_st_R2020a/Efficiency/LPF ==
  x : Inport
  Gain2 : Gain  Gain=2*pi*100
  Integrator1 : Integrator
  Sum : Sum  Inputs=+-
  xf : Outport
  wires:
  Integrator1/1 -> xf/1, Sum/2
  Sum/1 -> Gain2/1
  x/1 -> Sum/1
  Gain2/1 -> Integrator1/1

== system pmsm_model_Lab3_MTPA_st_R2020a/Efficiency/LPF  ==
  x : Inport
  Gain2 : Gain  Gain=2*pi*100
  Integrator1 : Integrator
  Sum : Sum  Inputs=+-
  xf : Outport
  wires:
  Gain2/1 -> Integrator1/1
  x/1 -> Sum/1
  Sum/1 -> Gain2/1
  Integrator1/1 -> xf/1, Sum/2

== system pmsm_model_Lab3_MTPA_st_R2020a/Efficiency/LPF   ==
  x : Inport
  Gain2 : Gain  Gain=2*pi*10
  Integrator1 : Integrator  InitialCondition=Pe0/1000
  Sum : Sum  Inputs=+-
  xf : Outport
  wires:
  Integrator1/1 -> xf/1, Sum/2
  Sum/1 -> Gain2/1
  x/1 -> Sum/1
  Gain2/1 -> Integrator1/1

== system pmsm_model_Lab3_MTPA_st_R2020a/Efficiency/LPF  1 ==
  x : Inport
  Gain2 : Gain  Gain=2*pi*1000
  Integrator1 : Integrator  InitialCondition=Pe0/1000
  Sum : Sum  Inputs=+-
  xf : Outport
  wires:
  Gain2/1 -> Integrator1/1
  x/1 -> Sum/1
  Sum/1 -> Gain2/1
  Integrator1/1 -> Sum/2, xf/1

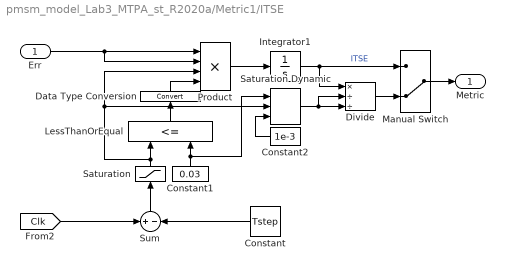
== system pmsm_model_Lab3_MTPA_st_R2020a/Metric1/ITSE ==
  Err : Inport
  Constant : Constant  Value=Tstep
  Constant1 : Constant  Value=0.03
  Constant2 : Constant  Value=1e-3
  Data Type Conversion : DataTypeConversion  SaturateOnIntegerOverflow=off  RndMeth=Floor
  Divide : Product  Inputs=*//
  Integrator1 : Integrator
  LessThanOrEqual : RelationalOperator  Operator=<=  OutDataTypeStr=boolean  RndMeth=Simplest  InputSameDT=off
  Manual Switch : ManualSwitch  CurrentSetting=0
  Product : Product  Inputs=4
  Saturation : Saturate  UpperLimit=inf  LowerLimit=0
  Saturation Dynamic : simulink/Discontinuities/Saturation Dynamic  OutMin=[]  OutMax=[]  OutDataTypeStr=Inherit: Same as second input  OutDataType=fixdt(1, 16)  OutScaling=2^-10  DoSatur=off
  Sum : Sum  Inputs=+|-
  Metric : Outport
  wires:
  Sum/1 -> Saturation/1
  Integrator1/1 -> Divide/1, Manual Switch/1  "ITSE"
  Err/1 -> Product/1, Product/2
  Product/1 -> Integrator1/1
  [Clk] -> Sum/1
  Saturation/1 -> Saturation Dynamic/2, Product/3, LessThanOrEqual/1
  Constant/1 -> Sum/2
  Divide/1 -> Manual Switch/2
  Manual Switch/1 -> Metric/1
  Saturation Dynamic/1 -> Divide/3, Divide/2
  LessThanOrEqual/1 -> Data Type Conversion/1
  Constant1/1 -> Saturation Dynamic/1, LessThanOrEqual/2
  Data Type Conversion/1 -> Product/4
  Constant2/1 -> Saturation Dynamic/3

== system pmsm_model_Lab3_MTPA_st_R2020a/Metric1/LPF ==
  x : Inport
  Gain : Gain  Gain=2*pi*10
  Integrator : Integrator
  Sum : Sum  Inputs=|+-
  xf : Outport
  wires:
  Gain/1 -> Integrator/1
  Sum/1 -> Gain/1
  Integrator/1 -> Sum/2, xf/1
  x/1 -> Sum/1

== system pmsm_model_Lab3_MTPA_st_R2020a/Metric1/RMSE ==
  Err : Inport
  Divide : Product  Inputs=*/
  Integrator1 : Integrator
  Integrator2 : Integrator
  Product : Product  Inputs=3
  Saturation : Saturate  UpperLimit=inf  LowerLimit=1e-3
  Sqrt : Sqrt
  Sqrt1 : Sqrt
  RMSE : Outport
  wires:
  Err/1 -> Product/1, Product/2
  Product/1 -> Integrator1/1
  Integrator1/1 -> Sqrt/1
  Sqrt/1 -> Divide/1
  [SS] -> Product/3, Integrator2/1
  Divide/1 -> RMSE/1
  Integrator2/1 -> Saturation/1
  Saturation/1 -> Sqrt1/1
  Sqrt1/1 -> Divide/2

== system pmsm_model_Lab3_MTPA_st_R2020a/Metric2/LPF ==
  Tm : Inport
  Gain : Gain  Gain=2*pi*10
  Integrator : Integrator  InitialCondition=Tm0
  Sum : Sum  Inputs=|+-
  Tav : Outport
  wires:
  Gain/1 -> Integrator/1
  Integrator/1 -> Tav/1, Sum/2
  Sum/1 -> Gain/1
  Tm/1 -> Sum/1

== system pmsm_model_Lab3_MTPA_st_R2020a/Metric2/Window ==
  "Tav " : Inport
  Dead Zone : DeadZone  LowerValue=-inf  UpperValue=Tstep
  Manual Switch : ManualSwitch
  Product : Product
  Tav : Outport
  wires:
  [SS] -> Manual Switch/1
  Dead Zone/1 -> Manual Switch/2  "ITSE"
  Manual Switch/1 -> Product/2
  Product/1 -> Tav/1
  [Clk] -> Dead Zone/1
  "Tav "/1 -> Product/1

== system pmsm_model_Lab3_MTPA_st_R2020a/Metric3/LPF ==
  Tm : Inport
  Gain : Gain  Gain=2*pi*30
  Integrator : Integrator  InitialCondition=Tm0
  Sum : Sum  Inputs=|+-
  Sum1 : Sum  Inputs=+-|
  Tmh : Outport
  Tm0 : Outport  Port=2
  wires:
  Tm/1 -> Sum1/1, Sum/1
  Integrator/1 -> Sum1/2, Tm0/1, Sum/2
  Sum/1 -> Gain/1
  Sum1/1 -> Tmh/1
  Gain/1 -> Integrator/1

== system pmsm_model_Lab3_MTPA_st_R2020a/Metric3/LPF2 ==
  x : Inport
  Gain : Gain  Gain=2*pi*10
  Integrator : Integrator
  Sum : Sum  Inputs=|+-
  xf : Outport
  wires:
  Gain/1 -> Integrator/1
  Sum/1 -> Gain/1
  Integrator/1 -> Sum/2, xf/1
  x/1 -> Sum/1

== system pmsm_model_Lab3_MTPA_st_R2020a/Metric3/Ripple ==
  Tmh : Inport
  Tm0 : Inport  Port=2
  Divide : Product  Inputs=*//
  Gain : Gain  Gain=100
  Integrator1 : Integrator
  Integrator2 : Integrator
  Product : Product  Inputs=3
  Saturation : Saturate  UpperLimit=inf  LowerLimit=1e-3
  Saturation1 : Saturate  UpperLimit=inf  LowerLimit=1e-3
  Sqrt : Sqrt
  Sqrt1 : Sqrt
  Ripple : Outport
  wires:
  Product/1 -> Integrator1/1
  Integrator1/1 -> Sqrt/1
  Sqrt/1 -> Divide/1
  [SS] -> Integrator2/1, Product/3
  Divide/1 -> Gain/1
  Gain/1 -> Ripple/1
  Integrator2/1 -> Saturation/1
  Saturation/1 -> Sqrt1/1
  Tm0/1 -> Saturation1/1
  Saturation1/1 -> Divide/3
  Sqrt1/1 -> Divide/2
  Tmh/1 -> Product/1, Product/2

== system pmsm_model_Lab3_MTPA_st_R2020a/PMSM/Flux_Current ==
  Psid : Inport
  Psiq : Inport  Port=2
  Id : Lookup_n-D  BreakpointsForDimension1=Psidv  BreakpointsForDimension2=Psiqv  Table=Idd  InternalRulePriority=Speed  RndMeth=Simplest
      settings: InputPortMap=u0,u1
  Iq : Lookup_n-D  BreakpointsForDimension1=Psidv  BreakpointsForDimension2=Psiqv  Table=Iqq  InternalRulePriority=Speed  RndMeth=Simplest
      settings: InputPortMap=u0,u1
  Saturation : Saturate  UpperLimit=max(Psidv)  LowerLimit=min(Psidv)
  Saturation1 : Saturate  UpperLimit=max(Psiqv)  LowerLimit=min(Psiqv)
  id : Outport
  iq : Outport  Port=2
  wires:
  Psiq/1 -> Saturation1/1
  Psid/1 -> Saturation/1
  Iq/1 -> iq/1
  Id/1 -> id/1
  Saturation/1 -> Iq/1, Id/1
  Saturation1/1 -> Iq/2, Id/2

== system pmsm_model_Lab3_MTPA_st_R2020a/PMSM/abc_dq ==
  abc : Inport
  sin_cos : Inport  Port=2
  Demux : Demux  Outputs=2
      settings: DisplayOption=none
  Demux1 : Demux  Outputs=2
      settings: DisplayOption=none
  Gain3 : Gain  Gain=C32inv  Multiplication=Matrix(K*u)  OutDataTypeStr=Inherit: Same as input  ParamDataTypeStr=Inherit: Same as input
  Mux : Mux  Inputs=2
  Product{,1..3} (4 alike) : Product  InputSameDT=on  RndMeth=Zero  SaturateOnIntegerOverflow=on  OutDataTypeStr=Inherit: Same as first input
  Sum : Sum  Inputs=|++  InputSameDT=on  SaturateOnIntegerOverflow=on  OutDataTypeStr=Inherit: Same as first input
  Sum1 : Sum  Inputs=|-+  InputSameDT=on  SaturateOnIntegerOverflow=on  OutDataTypeStr=Inherit: Same as first input
  dq : Outport
  wires:
  Sum1/1 -> Mux/2
  Mux/1 -> dq/1
  Demux1/1 -> Product2/2, Product1/2
  sin_cos/1 -> Demux1/1
  Demux/2 -> Product3/2, Product1/1
  Gain3/1 -> Demux/1  "alpha_beta"
  abc/1 -> Gain3/1
  Demux1/2 -> Product3/1, Product/2
  Demux/1 -> Product2/1, Product/1
  Sum/1 -> Mux/1
  Product3/1 -> Sum1/2
  Product2/1 -> Sum1/1
  Product1/1 -> Sum/2
  Product/1 -> Sum/1

== system pmsm_model_Lab3_MTPA_st_R2020a/PMSM/dq_abc ==
  dq : Inport
  sin_cos : Inport  Port=2
  Demux1 : Demux  Outputs=2
      settings: DisplayOption=none
  Demux2 : Demux  Outputs=2
      settings: DisplayOption=none
  Gain1 : Gain  Gain=C32  Multiplication=Matrix(K*u)  OutDataTypeStr=Inherit: Same as input  ParamDataTypeStr=Inherit: Same as input
  Mux : Mux  Inputs=2
  Product{,1..3} (4 alike) : Product  InputSameDT=on  RndMeth=Zero  SaturateOnIntegerOverflow=on  OutDataTypeStr=Inherit: Same as first input
  Sum : Sum  Inputs=|+-  InputSameDT=on  SaturateOnIntegerOverflow=on  OutDataTypeStr=Inherit: Same as first input
  Sum1 : Sum  Inputs=|++  InputSameDT=on  SaturateOnIntegerOverflow=on  OutDataTypeStr=Inherit: Same as first input
  abc : Outport
  wires:
  Mux/1 -> Gain1/1
  Demux1/1 -> Product2/2, Product1/2
  sin_cos/1 -> Demux1/1
  dq/1 -> Demux2/1
  Demux1/2 -> Product3/1, Product/2
  Product3/1 -> Sum1/2
  Product2/1 -> Sum1/1
  Product1/1 -> Sum/2
  Product/1 -> Sum/1
  Demux2/1 -> Product/1, Product2/1
  Demux2/2 -> Product3/2, Product1/1
  Sum/1 -> Mux/1
  Sum1/1 -> Mux/2
  Gain1/1 -> abc/1

== system pmsm_model_Lab3_MTPA_st_R2020a/PMSM/sin_cos ==
  thetae : Inport
  Mux1 : Mux  Inputs=2
  Trigonometric Function : Trigonometry
  Trigonometric Function1 : Trigonometry  Operator=cos
  sin_cos : Outport
  wires:
  Trigonometric Function/1 -> Mux1/1
  Trigonometric Function1/1 -> Mux1/2
  thetae/1 -> Trigonometric Function1/1, Trigonometric Function/1
  Mux1/1 -> sin_cos/1

== system pmsm_model_Lab3_MTPA_st_R2020a/SPWM/S1 ==
  "C " : Inport
  NOT : Logic  Operator=NOT  IconShape=distinctive  AllPortsSameDT=off  OutDataTypeStr=boolean
  C : Outport
  C* : Outport  Port=2
  wires:
  "C "/1 -> C/1, NOT/1
  NOT/1 -> C*/1

== system pmsm_model_Lab3_MTPA_st_R2020a/SPWM/S2 ==
  "C " : Inport
  NOT : Logic  Operator=NOT  IconShape=distinctive  AllPortsSameDT=off  OutDataTypeStr=boolean
  C : Outport
  C* : Outport  Port=2
  wires:
  NOT/1 -> C*/1
  "C "/1 -> NOT/1, C/1

== system pmsm_model_Lab3_MTPA_st_R2020a/SPWM/S3 ==
  "C " : Inport
  NOT : Logic  Operator=NOT  IconShape=distinctive  AllPortsSameDT=off  OutDataTypeStr=boolean
  C : Outport
  C* : Outport  Port=2
  wires:
  "C "/1 -> C/1, NOT/1
  NOT/1 -> C*/1

== system pmsm_model_Lab3_MTPA_st_R2020a/SPWM/carrier ==
  t : Inport
  Abs : Abs
  Constant2 : Constant  Value=-Vp
  Signal Generator : SignalGenerator  WaveForm=sawtooth  TimeSource=Use external signal  Amplitude=2*Vp  Frequency=1/Tp
  Sum2 : Sum  SaturateOnIntegerOverflow=on
  Vp : Outport
  wires:
  Sum2/1 -> Vp/1
  Constant2/1 -> Sum2/1
  Abs/1 -> Sum2/2
  Signal Generator/1 -> Abs/1
  t/1 -> Signal Generator/1

== system pmsm_model_Lab3_MTPA_st_R2020a/VSI/V1 ==
  C : Inport
  C* : Inport  Port=2
  I : Inport  Port=3
  Vs : Inport  Port=4
  Compare To Zero : simulink/Logic and Bit Operations/Compare To Zero  relop=>  OutDataTypeStr=boolean  ZeroCross=off
  Demux : Demux  Outputs=2
  Leg : CombinatorialLogic  TruthTable=[1 1;0 0;1 1;0.5 1;0 0;0 0;1 1;0.5 1]
  Mux : Mux  Inputs=3
  Product1 : Product  SaturateOnIntegerOverflow=on  OutDataTypeStr=Inherit: Same as first input
  Product3 : Product  SaturateOnIntegerOverflow=on  OutDataTypeStr=Inherit: Same as first input
  Sum1 : Sum  Inputs=-+|  SaturateOnIntegerOverflow=on
  Vdrop : Lookup_n-D  NumberOfTableDimensions=1  BreakpointsForDimension1=Idrop  Table=Vdrop  InternalRulePriority=Speed  RndMeth=Simplest
  V : Outport
  il : Outport  Port=2
  wires:
  Mux/1 -> Leg/1
  I/1 -> Product3/2, Vdrop/1, Compare To Zero/1
  C*/1 -> Mux/3
  C/1 -> Mux/2
  Compare To Zero/1 -> Mux/1
  Leg/1 -> Demux/1
  Demux/1 -> Product1/2
  Vs/1 -> Product1/1
  Sum1/1 -> V/1
  Product3/1 -> il/1
  Demux/2 -> Product3/1
  Product1/1 -> Sum1/2
  Vdrop/1 -> Sum1/1

== system pmsm_model_Lab3_MTPA_st_R2020a/VSI/V2 ==
  C : Inport
  C* : Inport  Port=2
  I : Inport  Port=3
  Vs : Inport  Port=4
  Compare To Zero : simulink/Logic and Bit Operations/Compare To Zero  relop=>  OutDataTypeStr=boolean  ZeroCross=off
  Demux : Demux  Outputs=2
  Leg : CombinatorialLogic  TruthTable=[1 1;0 0;1 1;0.5 1;0 0;0 0;1 1;0.5 1]
  Mux : Mux  Inputs=3
  Product1 : Product  SaturateOnIntegerOverflow=on  OutDataTypeStr=Inherit: Same as first input
  Product3 : Product  SaturateOnIntegerOverflow=on  OutDataTypeStr=Inherit: Same as first input
  Sum1 : Sum  Inputs=-+|  SaturateOnIntegerOverflow=on
  Vdrop : Lookup_n-D  NumberOfTableDimensions=1  BreakpointsForDimension1=Idrop  Table=Vdrop  InternalRulePriority=Speed  RndMeth=Simplest
  V : Outport
  il : Outport  Port=2
  wires:
  Vdrop/1 -> Sum1/1
  Product1/1 -> Sum1/2
  Demux/2 -> Product3/1
  Product3/1 -> il/1
  Sum1/1 -> V/1
  Vs/1 -> Product1/1
  Demux/1 -> Product1/2
  Leg/1 -> Demux/1
  Compare To Zero/1 -> Mux/1
  C/1 -> Mux/2
  C*/1 -> Mux/3
  I/1 -> Compare To Zero/1, Vdrop/1, Product3/2
  Mux/1 -> Leg/1

== system pmsm_model_Lab3_MTPA_st_R2020a/VSI/V3 ==
  C : Inport
  C* : Inport  Port=2
  I : Inport  Port=3
  Vs : Inport  Port=4
  Compare To Zero : simulink/Logic and Bit Operations/Compare To Zero  relop=>  OutDataTypeStr=boolean  ZeroCross=off
  Demux : Demux  Outputs=2
  Leg : CombinatorialLogic  TruthTable=[1 1;0 0;1 1;0.5 1;0 0;0 0;1 1;0.5 1]
  Mux : Mux  Inputs=3
  Product1 : Product  SaturateOnIntegerOverflow=on  OutDataTypeStr=Inherit: Same as first input
  Product3 : Product  SaturateOnIntegerOverflow=on  OutDataTypeStr=Inherit: Same as first input
  Sum1 : Sum  Inputs=-+|  SaturateOnIntegerOverflow=on
  Vdrop : Lookup_n-D  NumberOfTableDimensions=1  BreakpointsForDimension1=Idrop  Table=Vdrop  InternalRulePriority=Speed  RndMeth=Simplest
  V : Outport
  il : Outport  Port=2
  wires:
  Mux/1 -> Leg/1
  I/1 -> Product3/2, Vdrop/1, Compare To Zero/1
  C*/1 -> Mux/3
  C/1 -> Mux/2
  Compare To Zero/1 -> Mux/1
  Leg/1 -> Demux/1
  Demux/1 -> Product1/2
  Vs/1 -> Product1/1
  Sum1/1 -> V/1
  Product3/1 -> il/1
  Demux/2 -> Product3/1
  Product1/1 -> Sum1/2
  Vdrop/1 -> Sum1/1

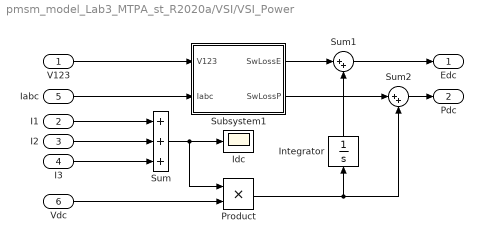
== system pmsm_model_Lab3_MTPA_st_R2020a/VSI/VSI_Power ==
  V123 : Inport
  I1 : Inport  Port=2
  I2 : Inport  Port=3
  I3 : Inport  Port=4
  Iabc : Inport  Port=5
  Vdc : Inport  Port=6
  Idc : Scope
  Integrator : Integrator
  Product : Product
  Subsystem1 : Subsystem
  Sum : Sum  Inputs=+++
  Sum1 : Sum  Inputs=|++
  Sum2 : Sum  Inputs=|++
  Edc : Outport
  Pdc : Outport  Port=2
  wires:
  Product/1 -> Sum2/2, Integrator/1
  V123/1 -> Subsystem1/1(V123)
  Sum/1 -> Product/1, Idc/1
  I1/1 -> Sum/1
  Subsystem1/2(SwLossP) -> Sum2/1
  I2/1 -> Sum/2
  Integrator/1 -> Sum1/2
  I3/1 -> Sum/3
  Vdc/1 -> Product/2
  Sum1/1 -> Edc/1
  Sum2/1 -> Pdc/1
  Iabc/1 -> Subsystem1/2(Iabc)
  Subsystem1/1(SwLossE) -> Sum1/1

== system pmsm_model_Lab3_MTPA_st_R2020a/Control/dq_abc/DutyCycles ==
  VDC : Inport
  Vabc* : Inport  Port=2
  Constant : Constant  Value=0.5
  Divide : Product  Inputs=*/
  Gain : Gain  Gain=0.5*0.9925
  Gain1 : Gain  Gain=-1
  Saturation Dynamic : simulink/Discontinuities/Saturation Dynamic  OutMin=[]  OutMax=[]  OutDataTypeStr=Inherit: Same as second input  OutDataType=fixdt(1, 16)  OutScaling=2^-10  DoSatur=off
  Sum : Sum  Inputs=|++
  dabc* : Outport
  wires:
  Divide/1 -> Sum/1
  Sum/1 -> dabc*/1
  Constant/1 -> Sum/2
  VDC/1 -> Gain/1, Divide/2
  Saturation Dynamic/1 -> Divide/1
  Vabc*/1 -> Saturation Dynamic/2
  Gain/1 -> Gain1/1, Saturation Dynamic/1
  Gain1/1 -> Saturation Dynamic/3

== system pmsm_model_Lab3_MTPA_st_R2020a/Control/dq_abc/THIPWM ==
  Vabc* : Inport
  Add : Sum
  Add1 : Sum
  Gain : Gain  Gain=-0.5
  Manual Switch : ManualSwitch
  MinMax1 : MinMax  InputSameDT=on  SaturateOnIntegerOverflow=on
  MinMax2 : MinMax  Function=max  InputSameDT=on  SaturateOnIntegerOverflow=on
  Vabc3* : Outport
  wires:
  Vabc*/1 -> MinMax2/1, MinMax1/1, Manual Switch/2, Add1/2
  MinMax2/1 -> Add/2
  Add/1 -> Gain/1
  Gain/1 -> Add1/1
  Add1/1 -> Manual Switch/1
  MinMax1/1 -> Add/1
  Manual Switch/1 -> Vabc3*/1

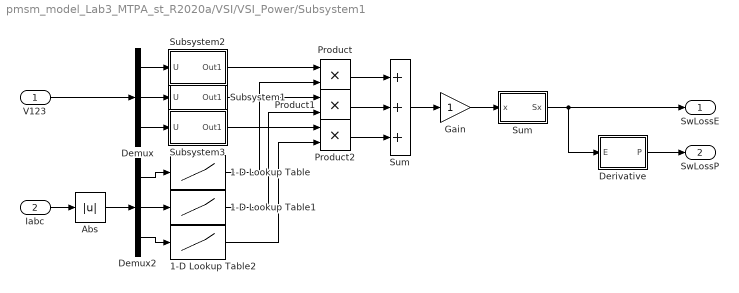
== system pmsm_model_Lab3_MTPA_st_R2020a/VSI/VSI_Power/Subsystem1 ==
  V123 : Inport
  Iabc : Inport  Port=2
  1-D Lookup Table : Lookup_n-D  NumberOfTableDimensions=1  BreakpointsForDimension1=Isw  Table=SwLoss  InternalRulePriority=Speed  RndMeth=Simplest
  1-D Lookup Table1 : Lookup_n-D  NumberOfTableDimensions=1  BreakpointsForDimension1=Isw  Table=SwLoss  InternalRulePriority=Speed  RndMeth=Simplest
  1-D Lookup Table2 : Lookup_n-D  NumberOfTableDimensions=1  BreakpointsForDimension1=Isw  Table=SwLoss  InternalRulePriority=Speed  RndMeth=Simplest
  Abs : Abs  SaturateOnIntegerOverflow=off
  Demux : Demux  Outputs=3
  Demux2 : Demux  Outputs=3
  Derivative : Subsystem
  Gain : Gain
  Product : Product
  Product1 : Product
  Product2 : Product
  Subsystem1 : Subsystem
  Subsystem2 : Subsystem
  Subsystem3 : Subsystem
  Sum : Sum  Inputs=+++
  "Sum " : Subsystem
  SwLossE : Outport
  SwLossP : Outport  Port=2
  wires:
  V123/1 -> Demux/1
  Abs/1 -> Demux2/1
  Demux2/3 -> 1-D Lookup Table2/1
  Demux2/2 -> 1-D Lookup Table1/1
  Demux2/1 -> 1-D Lookup Table/1
  Product2/1 -> Sum/3
  Product1/1 -> Sum/2
  Product/1 -> Sum/1
  Subsystem1/1(Out1) -> Product1/1
  Subsystem3/1(Out1) -> Product2/1
  Iabc/1 -> Abs/1
  Sum/1 -> Gain/1
  Subsystem2/1(Out1) -> Product/1
  Demux/3 -> Subsystem3/1(U)
  Demux/2 -> Subsystem1/1(U)
  Demux/1 -> Subsystem2/1(U)
  1-D Lookup Table/1 -> Product/2
  1-D Lookup Table1/1 -> Product1/2
  1-D Lookup Table2/1 -> Product2/2
  Derivative/1(P) -> SwLossP/1
  "Sum "/1(Sx) -> Derivative/1(E), SwLossE/1
  Gain/1 -> "Sum "/1(x)

== system pmsm_model_Lab3_MTPA_st_R2020a/VSI/VSI_Power/Subsystem1/Derivative ==
  E : Inport
  Divide1 : Product  Inputs=/*
  Saturation : Saturate  UpperLimit=inf  LowerLimit=1e-9
  Sum2 : Sum  Inputs=|+-
  Sum5 : Sum  Inputs=+-|
  Unit Delay1 : UnitDelay  SampleTime=-1  HasFrameUpgradeWarning=on
  Unit Delay2 : UnitDelay  SampleTime=-1  HasFrameUpgradeWarning=on
  P : Outport
  wires:
  Unit Delay2/1 -> Sum5/2
  Saturation/1 -> Divide1/1
  [Clk] -> Sum5/1, Unit Delay2/1
  E/1 -> Unit Delay1/1, Sum2/1
  Unit Delay1/1 -> Sum2/2
  Sum5/1 -> Saturation/1
  Sum2/1 -> Divide1/2
  Divide1/1 -> P/1

== system pmsm_model_Lab3_MTPA_st_R2020a/VSI/VSI_Power/Subsystem1/Subsystem1 ==
  U : Inport
  Gain : Gain
  Gain1 : Gain
  Subsystem : Subsystem
  Subsystem1 : Subsystem
  Sum3 : Sum  Inputs=|++  SaturateOnIntegerOverflow=on
  Out1 : Outport
  wires:
  U/1 -> Subsystem/1(U), Subsystem1/1(U)
  Subsystem1/1(Out1) -> Gain1/1
  Subsystem/1(Out1) -> Gain/1
  Gain/1 -> Sum3/2
  Sum3/1 -> Out1/1
  Gain1/1 -> Sum3/1

== system pmsm_model_Lab3_MTPA_st_R2020a/VSI/VSI_Power/Subsystem1/Subsystem2 ==
  U : Inport
  Gain : Gain
  Gain1 : Gain
  Subsystem : Subsystem
  Subsystem1 : Subsystem
  Sum3 : Sum  Inputs=|++  SaturateOnIntegerOverflow=on
  Out1 : Outport
  wires:
  Gain1/1 -> Sum3/1
  Sum3/1 -> Out1/1
  Gain/1 -> Sum3/2
  Subsystem/1(Out1) -> Gain/1
  Subsystem1/1(Out1) -> Gain1/1
  U/1 -> Subsystem1/1(U), Subsystem/1(U)

== system pmsm_model_Lab3_MTPA_st_R2020a/VSI/VSI_Power/Subsystem1/Subsystem3 ==
  U : Inport
  Gain : Gain
  Gain1 : Gain
  Subsystem : Subsystem
  Subsystem1 : Subsystem
  Sum3 : Sum  Inputs=|++  SaturateOnIntegerOverflow=on
  Out1 : Outport
  wires:
  Gain1/1 -> Sum3/1
  Sum3/1 -> Out1/1
  Gain/1 -> Sum3/2
  Subsystem/1(Out1) -> Gain/1
  Subsystem1/1(Out1) -> Gain1/1
  U/1 -> Subsystem1/1(U), Subsystem/1(U)

== system pmsm_model_Lab3_MTPA_st_R2020a/VSI/VSI_Power/Subsystem1/Sum  ==
  x : Inport
  Memory : Memory
  Sum1 : Sum  Inputs=|++
  Sx : Outport
  wires:
  Memory/1 -> Sum1/2
  x/1 -> Sum1/1
  Sum1/1 -> Memory/1, Sx/1

== system pmsm_model_Lab3_MTPA_st_R2020a/VSI/VSI_Power/Subsystem1/Subsystem1/Subsystem ==
  U : Inport
  Compare To Constant : simulink/Logic and Bit Operations/Compare To Constant  relop=<  const=-VDC0  OutDataTypeStr=uint8
  Memory : Memory
  Sum : Sum  Inputs=+-|
  Out1 : Outport
  wires:
  Compare To Constant/1 -> Out1/1
  U/1 -> Sum/1, Memory/1
  Sum/1 -> Compare To Constant/1
  Memory/1 -> Sum/2

== system pmsm_model_Lab3_MTPA_st_R2020a/VSI/VSI_Power/Subsystem1/Subsystem1/Subsystem1 ==
  U : Inport
  Compare To Constant : simulink/Logic and Bit Operations/Compare To Constant  relop=>  const=VDC0  OutDataTypeStr=uint8
  Memory : Memory
  Sum : Sum  Inputs=+-|
  Out1 : Outport
  wires:
  Compare To Constant/1 -> Out1/1
  Memory/1 -> Sum/2
  Sum/1 -> Compare To Constant/1
  U/1 -> Sum/1, Memory/1

== system pmsm_model_Lab3_MTPA_st_R2020a/VSI/VSI_Power/Subsystem1/Subsystem2/Subsystem ==
  U : Inport
  Compare To Constant : simulink/Logic and Bit Operations/Compare To Constant  relop=<  const=-VDC0  OutDataTypeStr=uint8
  Memory : Memory
  Sum : Sum  Inputs=+-|
  Out1 : Outport
  wires:
  Memory/1 -> Sum/2
  Sum/1 -> Compare To Constant/1
  U/1 -> Memory/1, Sum/1
  Compare To Constant/1 -> Out1/1
